simulink model "Rebuild"  (R2024b)
settings: Solver=VariableStepAuto  StartTime=0.0  StopTime=12  RelTol=1e-3
values from neighbouring files (symbols this model uses):
  A = 1.1    [RT14e_Parameters.m]    (also in RT15e_Parameters.m = 1.088; RT15evo_Parameters.m = 1.088)
  Aero_balance = 55    [RT14e_Parameters.m]    (also in RT15e_Parameters.m; RT15evo_Parameters.m)
  Aeromaps_ON = 0    [SIM_setup.m]
  air_density = 1.2    [SIM_setup.m]
  Balance_FW = Data_FW_STD(1:end,2)    [RT15e_Parameters.m]    (also in RT15evo_Parameters.m)
  Balance_R_11 = Data_R_11(1:end,2)    [RT15e_Parameters.m]    (also in RT15evo_Parameters.m)
  Br_coef_of_friction_F = 0.33    [RT14e_Parameters.m]    (also in RT15e_Parameters.m; RT15evo_Parameters.m)
  Br_coef_of_friction_R = 0.33    [RT14e_Parameters.m]    (also in RT15e_Parameters.m; RT15evo_Parameters.m)
  Br_pistons_area_F = 3617.26/1e6    (= 0.00361726)    [RT14e_Parameters.m]    (also in RT15e_Parameters.m; RT15evo_Parameters.m)
  Br_pistons_area_R = 2026.83/1e6    (= 0.00202683)    [RT14e_Parameters.m]    (also in RT15e_Parameters.m; RT15evo_Parameters.m)
  CdA = 1.31*A    (= 1.441)    [RT14e_Parameters.m]    (also in RT15e_Parameters.m = 1.700544; RT15evo_Parameters.m = 1.700544)
  CdA_FW = Data_FW_STD(1:end,3)    [RT15e_Parameters.m]    (also in RT15evo_Parameters.m)
  CdA_R_11 = Data_R_11(1:end,3)    [RT15e_Parameters.m]    (also in RT15evo_Parameters.m)
  ClA = 3.3*A    (= 3.63)    [RT14e_Parameters.m]    (also in RT15e_Parameters.m = 4.36288; RT15evo_Parameters.m = 4.36288)
  ClA_FW = Data_FW_STD(1:end,4)    [RT15e_Parameters.m]    (also in RT15evo_Parameters.m)
  ClA_R_11 = Data_R_11(1:end,4)    [RT15e_Parameters.m]    (also in RT15evo_Parameters.m)
  CoG_z = 0.35    [RT14e_Parameters.m]    (also in RT15e_Parameters.m = 0.28495; RT15evo_Parameters.m = 0.28495)
  Default_Fz_FL = Default_Fz_F/2 + (Default_Fz_F*CoG_y/Track_Front)    [RT14e_Parameters.m]    (also in RT15e_Parameters.m; RT15evo_Parameters.m)
  Default_Fz_FR = Default_Fz_F/2 - (Default_Fz_F*CoG_y/Track_Front)    [RT14e_Parameters.m]    (also in RT15e_Parameters.m; RT15evo_Parameters.m)
  Default_Fz_RL = Default_Fz_R/2 + (Default_Fz_R*CoG_y/Track_Rear)    [RT14e_Parameters.m]    (also in RT15e_Parameters.m; RT15evo_Parameters.m)
  Default_Fz_RR = Default_Fz_R/2 - (Default_Fz_R*CoG_y/Track_Rear)    [RT14e_Parameters.m]    (also in RT15e_Parameters.m; RT15evo_Parameters.m)
  Effective_br_disk_r_F = 0.0905    [RT14e_Parameters.m]    (also in RT15e_Parameters.m; RT15evo_Parameters.m)
  Effective_br_disk_r_R = 0.0895    [RT14e_Parameters.m]    (also in RT15e_Parameters.m; RT15evo_Parameters.m)
  Front_brake_balance = 0.0    (= 0)    [RT14e_Parameters.m]    (also in RT15e_Parameters.m; RT15evo_Parameters.m)
  Front_brake_pump_area = 153.94    [RT14e_Parameters.m]    (also in RT15e_Parameters.m; RT15evo_Parameters.m)
  Front_desired_brake_p_balance = 0.6    [RT14e_Parameters.m]    (also in RT15e_Parameters.m; RT15evo_Parameters.m)
  FW_Setup = Data_FW_STD(1:end,1)    [RT15e_Parameters.m]    (also in RT15evo_Parameters.m)
  Fx = Data_Fx(2:end,3:end)    [RT14e_Parameters.m]    (also in RT15e_Parameters.m; RT15evo_Parameters.m)
  Fy = Data_Fy(2:end,3:end)    [RT14e_Parameters.m]    (also in RT15e_Parameters.m; RT15evo_Parameters.m)
  Fz = Data_Fy(2:end,2)    [RT14e_Parameters.m]    (also in RT15e_Parameters.m; RT15evo_Parameters.m)
  g = 9.81    [SIM_setup.m]
  Gear_ratio = 12.9    [RT14e_Parameters.m]    (also in RT15e_Parameters.m; RT15evo_Parameters.m)
  Iz_wehicle = 120    [RT14e_Parameters.m]    (also in RT15e_Parameters.m; RT15evo_Parameters.m)
  Iz_wheel = 0.15    [RT14e_Parameters.m]    (also in RT15e_Parameters.m; RT15evo_Parameters.m)
  Lf = Wheelbase - CoG_x    (= 0.77)    [RT14e_Parameters.m]    (also in RT15e_Parameters.m = 0.7504; RT15evo_Parameters.m = 0.7504)
  LLTD = 0.45    [RT14e_Parameters.m]    (also in RT15e_Parameters.m = 0.55; RT15evo_Parameters.m = 0.55)
  Lock_brake_balance = false    [RT14e_Parameters.m]    (also in RT15e_Parameters.m; RT15evo_Parameters.m)
  Lr = Wheelbase - Lf    (= 0.755)    [RT14e_Parameters.m]    (also in RT15e_Parameters.m = 0.7746; RT15evo_Parameters.m = 0.7746)
  Mass = Vehicle_mass + Driver_mass    (= 290)    [RT14e_Parameters.m]    (also in RT15e_Parameters.m = 265; RT15evo_Parameters.m)
  Motor_maximum_power = 35366    [RT14e_Parameters.m]    (also in RT15e_Parameters.m; RT15evo_Parameters.m)
  RB_torque_setting_1 = -2    [RT14e_Parameters.m]    (also in RT15e_Parameters.m; RT15evo_Parameters.m)
  RB_torque_setting_10 = -20    [RT14e_Parameters.m]    (also in RT15e_Parameters.m; RT15evo_Parameters.m)
  RB_torque_setting_2 = -4    [RT14e_Parameters.m]    (also in RT15e_Parameters.m; RT15evo_Parameters.m)
  RB_torque_setting_3 = -6    [RT14e_Parameters.m]    (also in RT15e_Parameters.m; RT15evo_Parameters.m)
  RB_torque_setting_4 = -8    [RT14e_Parameters.m]    (also in RT15e_Parameters.m; RT15evo_Parameters.m)
  RB_torque_setting_5 = -10    [RT14e_Parameters.m]    (also in RT15e_Parameters.m; RT15evo_Parameters.m)
  RB_torque_setting_6 = -12    [RT14e_Parameters.m]    (also in RT15e_Parameters.m; RT15evo_Parameters.m)
  RB_torque_setting_7 = -14    [RT14e_Parameters.m]    (also in RT15e_Parameters.m; RT15evo_Parameters.m)
  RB_torque_setting_8 = -16    [RT14e_Parameters.m]    (also in RT15e_Parameters.m; RT15evo_Parameters.m)
  RB_torque_setting_9 = -18    [RT14e_Parameters.m]    (also in RT15e_Parameters.m; RT15evo_Parameters.m)
  Rear_brake_pump_area = 198.56    [RT14e_Parameters.m]    (also in RT15e_Parameters.m; RT15evo_Parameters.m)
  Roll_Angle_11 = Data_R_11(1:end,1)    [RT15e_Parameters.m]    (also in RT15evo_Parameters.m)
  SA = Data_Fy(1,3:end)    [RT14e_Parameters.m]    (also in RT15e_Parameters.m; RT15evo_Parameters.m)
  SR = Data_Fx(1,3:end)    [RT14e_Parameters.m]    (also in RT15e_Parameters.m; RT15evo_Parameters.m)
  start_acc_x = double(start_acc_x_ts.Data)    [SIM_setup.m]
  start_acc_y = double(start_acc_y_ts.Data)    [SIM_setup.m]
  start_time = 1188    [SIM_setup.m]
  start_velocity_x = double(start_velocity_x_ts.Data)    [SIM_setup.m]
  start_velocity_y = double(start_velocity_y_ts.Data)    [SIM_setup.m]
  start_yaw_acc = double(start_yaw_acc_ts.Data)    [SIM_setup.m]
  start_yaw_rate = double(start_yaw_rate_ts.Data)    [SIM_setup.m]
  Static_Camber_FL = 0    [RT14e_Parameters.m]    (also in RT15e_Parameters.m; RT15evo_Parameters.m)
  Static_Camber_FR = 0    [RT14e_Parameters.m]    (also in RT15e_Parameters.m; RT15evo_Parameters.m)
  Static_Camber_RL = 0    [RT14e_Parameters.m]    (also in RT15e_Parameters.m; RT15evo_Parameters.m)
  Static_Camber_RR = 0    [RT14e_Parameters.m]    (also in RT15e_Parameters.m; RT15evo_Parameters.m)
  Static_Toe_FL = 0    [RT14e_Parameters.m]    (also in RT15e_Parameters.m; RT15evo_Parameters.m)
  Static_Toe_FR = 0    [RT14e_Parameters.m]    (also in RT15e_Parameters.m; RT15evo_Parameters.m)
  Static_Toe_RL = 0    [RT14e_Parameters.m]    (also in RT15e_Parameters.m; RT15evo_Parameters.m)
  Static_Toe_RR = 0    [RT14e_Parameters.m]    (also in RT15e_Parameters.m; RT15evo_Parameters.m)
  Steering_Angle_FL = Data_Steering(1:end,2)    [RT14e_Parameters.m]    (also in RT15e_Parameters.m; RT15evo_Parameters.m)
  Steering_Angle_FR = Data_Steering(1:end,3)    [RT14e_Parameters.m]    (also in RT15e_Parameters.m; RT15evo_Parameters.m)
  Steering_Wheel_Angle = Data_Steering(1:end,1)    [RT14e_Parameters.m]    (also in RT15e_Parameters.m; RT15evo_Parameters.m)
  Tire_radius = 0.203    [RT14e_Parameters.m]    (also in RT15e_Parameters.m; RT15evo_Parameters.m)
  Torque_limit_2 = Motor_maximum_torque*0.2    (= 5.82)    [RT14e_Parameters.m]    (also in RT15e_Parameters.m; RT15evo_Parameters.m)
  Torque_limit_3 = Motor_maximum_torque*0.3    (= 8.73)    [RT14e_Parameters.m]    (also in RT15e_Parameters.m; RT15evo_Parameters.m)
  Torque_limit_4 = Motor_maximum_torque*0.4    (= 11.64)    [RT14e_Parameters.m]    (also in RT15e_Parameters.m; RT15evo_Parameters.m)
  Torque_limit_5 = Motor_maximum_torque*0.5    (= 14.55)    [RT14e_Parameters.m]    (also in RT15e_Parameters.m; RT15evo_Parameters.m)
  Torque_limit_6 = Motor_maximum_torque*0.6    (= 17.46)    [RT14e_Parameters.m]    (also in RT15e_Parameters.m; RT15evo_Parameters.m)
  Torque_limit_7 = Motor_maximum_torque*0.7    (= 20.37)    [RT14e_Parameters.m]    (also in RT15e_Parameters.m; RT15evo_Parameters.m)
  Torque_limit_8 = Motor_maximum_torque*0.8    (= 23.28)    [RT14e_Parameters.m]    (also in RT15e_Parameters.m; RT15evo_Parameters.m)
  Torque_limit_9 = 29.1    [RT14e_Parameters.m]    (also in RT15e_Parameters.m; RT15evo_Parameters.m)
  Torque_limit_max = Motor_maximum_torque    (= 29.1)    [RT14e_Parameters.m]    (also in RT15e_Parameters.m; RT15evo_Parameters.m)
  Torque_limit_min = Motor_maximum_torque*0.1    (= 2.91)    [RT14e_Parameters.m]    (also in RT15e_Parameters.m; RT15evo_Parameters.m)
  Torque_limit_set = 10    [RT14e_Parameters.m]    (also in RT15e_Parameters.m; RT15evo_Parameters.m)
  Track_Front = 1.2    [RT14e_Parameters.m]    (also in RT15e_Parameters.m; RT15evo_Parameters.m)
  Track_Rear = 1.18    [RT14e_Parameters.m]    (also in RT15e_Parameters.m; RT15evo_Parameters.m)
  TV_ON = 0    [SIM_setup.m]
  TV_RB_understeer_gradient_1 = -0.5    [RT14e_Parameters.m]    (also in RT15e_Parameters.m; RT15evo_Parameters.m)
  TV_RB_understeer_gradient_10 = 0.005    [RT14e_Parameters.m]    (also in RT15e_Parameters.m; RT15evo_Parameters.m)
  TV_RB_understeer_gradient_2 = -0.1    [RT14e_Parameters.m]    (also in RT15e_Parameters.m; RT15evo_Parameters.m)
  TV_RB_understeer_gradient_3 = 0.08    [RT14e_Parameters.m]    (also in RT15e_Parameters.m; RT15evo_Parameters.m)
  TV_RB_understeer_gradient_4 = 0.06    [RT14e_Parameters.m]    (also in RT15e_Parameters.m; RT15evo_Parameters.m)
  TV_RB_understeer_gradient_5 = 0.05    [RT14e_Parameters.m]    (also in RT15e_Parameters.m; RT15evo_Parameters.m)
  TV_RB_understeer_gradient_6 = 0.04    [RT14e_Parameters.m]    (also in RT15e_Parameters.m; RT15evo_Parameters.m)
  TV_RB_understeer_gradient_7 = 0.03    [RT14e_Parameters.m]    (also in RT15e_Parameters.m; RT15evo_Parameters.m)
  TV_RB_understeer_gradient_8 = 0.02    [RT14e_Parameters.m]    (also in RT15e_Parameters.m; RT15evo_Parameters.m)
  TV_RB_understeer_gradient_9 = 0.01    [RT14e_Parameters.m]    (also in RT15e_Parameters.m; RT15evo_Parameters.m)
  TV_understeer_gradient_1 = -0.5    [RT14e_Parameters.m]    (also in RT15e_Parameters.m; RT15evo_Parameters.m)
  TV_understeer_gradient_10 = 0.002    [RT14e_Parameters.m]    (also in RT15e_Parameters.m; RT15evo_Parameters.m)
  TV_understeer_gradient_2 = -0.1    [RT14e_Parameters.m]    (also in RT15e_Parameters.m; RT15evo_Parameters.m)
  TV_understeer_gradient_3 = 0.06    [RT14e_Parameters.m]    (also in RT15e_Parameters.m; RT15evo_Parameters.m)
  TV_understeer_gradient_4 = 0.05    [RT14e_Parameters.m]    (also in RT15e_Parameters.m; RT15evo_Parameters.m)
  TV_understeer_gradient_5 = 0.04    [RT14e_Parameters.m]    (also in RT15e_Parameters.m; RT15evo_Parameters.m)
  TV_understeer_gradient_6 = 0.03    [RT14e_Parameters.m]    (also in RT15e_Parameters.m; RT15evo_Parameters.m)
  TV_understeer_gradient_7 = 0.02    [RT14e_Parameters.m]    (also in RT15e_Parameters.m; RT15evo_Parameters.m)
  TV_understeer_gradient_8 = 0.01    [RT14e_Parameters.m]    (also in RT15e_Parameters.m; RT15evo_Parameters.m)
  TV_understeer_gradient_9 = 0.005    [RT14e_Parameters.m]    (also in RT15e_Parameters.m; RT15evo_Parameters.m)
  Vx_APPS_ON = 1    [SIM_setup.m]
  Wheel_rolling_resistance = 0.055    [RT14e_Parameters.m]    (also in RT15e_Parameters.m; RT15evo_Parameters.m)
  Wheelbase = 1.525    [RT14e_Parameters.m]    (also in RT15e_Parameters.m; RT15evo_Parameters.m)
undefined symbols (not defined in the file or in its folder): Actual_Torque_Value_RL, Actual_Torque_Value_RR, aero_balance, APPS, Brake_Pressure_Front, Brake_Pressure_Rear, Cl, lateral_load_transfer_distribution, maths_GPS_Velocity, Max_Torque, rad, s, Steering_position, tire_radius, wheel_base, Wheel_Speed_RL, Wheel_Speed_RR, Xsens_MTI_670_accX, Xsens_MTI_670_accY, Xsens_MTI_670_gyrZ
libraries: simulink x30, simulink_extras x11, slpidlib x9, dspstat3 x4, slrealtimeloglib x1, aerolibconvert2 x1
(part 2 of 6)

== system Rebuild/Main/Wheels & Tires/Fx ==
  Slips : Inport
  2-D Lookup Table1 : Lookup_n-D  BreakpointsForDimension1=Fz  BreakpointsForDimension2=SR  Table=Fx  UseLastTableValue=on  ApplyAccurateEfficientRounding=on  InternalRulePriority=Speed  RndMeth=Simplest
      settings: InputPortMap=u0,u1
  2-D Lookup Table2 : Lookup_n-D  BreakpointsForDimension1=Fz  BreakpointsForDimension2=SR  Table=Fx  UseLastTableValue=on  ApplyAccurateEfficientRounding=on  InternalRulePriority=Speed  RndMeth=Simplest
      settings: InputPortMap=u0,u1
  2-D Lookup Table3 : Lookup_n-D  BreakpointsForDimension1=Fz  BreakpointsForDimension2=SR  Table=Fx  ExtrapMethod=Clip  UseLastTableValue=on  ApplyAccurateEfficientRounding=on  InternalRulePriority=Speed  RndMeth=Simplest
      settings: InputPortMap=u0,u1
  2-D Lookup Table4 : Lookup_n-D  BreakpointsForDimension1=Fz  BreakpointsForDimension2=SR  Table=Fx  ExtrapMethod=Clip  UseLastTableValue=on  ApplyAccurateEfficientRounding=on  InternalRulePriority=Speed  RndMeth=Simplest
      settings: InputPortMap=u0,u1
  Bus Creator : BusCreator  Inputs=4
  Bus Selector : BusSelector  OutputSignals=Slip Ratio.Slip Ratio FL
  Bus Selector1 : BusSelector  OutputSignals=Tire Forces [N[.Fz [N].Fz FL [N]
  Bus Selector2 : BusSelector  OutputSignals=Slip Ratio.Slip Ratio FR
  Bus Selector3 : BusSelector  OutputSignals=Tire Forces [N[.Fz [N].Fz FR [N]
  Bus Selector4 : BusSelector  OutputSignals=Slip Ratio.Slip Ratio RL
  Bus Selector5 : BusSelector  OutputSignals=Tire Forces [N[.Fz [N].Fz RL [N]
  Bus Selector6 : BusSelector  OutputSignals=Slip Ratio.Slip Ratio RR
  Bus Selector7 : BusSelector  OutputSignals=Tire Forces [N[.Fz [N].Fz RR [N]
  Gain{,1..3} (4 alike) : Gain
  Fx [N] : Outport
  wires:
  2-D Lookup Table1/1 -> Gain/1  "Fx FL [N]"
  2-D Lookup Table2/1 -> Gain1/1  "Fx FR [N]"
  2-D Lookup Table3/1 -> Gain2/1  "Fx RL [N]"
  2-D Lookup Table4/1 -> Gain3/1  "Fx RR [N]"
  Bus Creator/1 -> Fx [N]/1  "Fx [N]"
  Slips/1 -> Bus Selector/1, Bus Selector6/1, Bus Selector4/1, Bus Selector2/1
  [Tires] -> Bus Selector1/1, Bus Selector7/1, Bus Selector5/1, Bus Selector3/1
  Bus Selector/1 -> 2-D Lookup Table1/2  "<Slip Ratio FL>"
  Bus Selector1/1 -> 2-D Lookup Table1/1  "<Fz FL [N]>"
  Bus Selector3/1 -> 2-D Lookup Table2/1  "<Fz FR [N]>"
  Bus Selector2/1 -> 2-D Lookup Table2/2  "<Slip Ratio FR>"
  Bus Selector5/1 -> 2-D Lookup Table3/1  "<Fz RL [N]>"
  Bus Selector4/1 -> 2-D Lookup Table3/2  "<Slip Ratio RL>"
  Bus Selector7/1 -> 2-D Lookup Table4/1  "<Fz RR [N]>"
  Bus Selector6/1 -> 2-D Lookup Table4/2  "<Slip Ratio RR>"
  Gain/1 -> Bus Creator/1  "Fx FL [N]"
  Gain1/1 -> Bus Creator/2  "Fx FR [N]"
  Gain2/1 -> Bus Creator/3  "Fx RL [N]"
  Gain3/1 -> Bus Creator/4  "Fx RR [N]"

== system Rebuild/Main/Wheels & Tires/Fy ==
  Slips : Inport
  2-D Lookup Table{,1..3} (4 alike) : Lookup_n-D  BreakpointsForDimension1=Fz  BreakpointsForDimension2=SA  Table=Fy  ExtrapMethod=Clip  UseLastTableValue=on  ApplyAccurateEfficientRounding=on  InternalRulePriority=Speed  RndMeth=Simplest
      settings: InputPortMap=u0,u1
  Bus Creator : BusCreator  Inputs=4
  Bus Selector : BusSelector  OutputSignals=Slip Angle [deg].Slip Angle FL [deg]
  Bus Selector1 : BusSelector  OutputSignals=Tire Forces [N[.Fz [N].Fz FL [N]
  Bus Selector2 : BusSelector  OutputSignals=Slip Angle [deg].Slip Angle FR [deg]
  Bus Selector3 : BusSelector  OutputSignals=Tire Forces [N[.Fz [N].Fz FR [N]
  Bus Selector4 : BusSelector  OutputSignals=Slip Angle [deg].Slip Angle RL [deg]
  Bus Selector5 : BusSelector  OutputSignals=Tire Forces [N[.Fz [N].Fz RL [N]
  Bus Selector6 : BusSelector  OutputSignals=Slip Angle [deg].Slip Angle RR [deg]
  Bus Selector7 : BusSelector  OutputSignals=Tire Forces [N[.Fz [N].Fz RR [N]
  Gain{,1..3} (4 alike) : Gain
  Fy [N] : Outport
  wires:
  2-D Lookup Table/1 -> Gain3/1  "Fy FL [N]"
  2-D Lookup Table1/1 -> Gain2/1  "Fy FR [N]"
  2-D Lookup Table3/1 -> Gain1/1  "Fy RL [N]"
  2-D Lookup Table2/1 -> Gain/1  "Fy RR [N]"
  Bus Creator/1 -> Fy [N]/1  "Fy [N]"
  Bus Selector2/1 -> 2-D Lookup Table1/2  "<Slip Angle FR [deg]>"
  Bus Selector3/1 -> 2-D Lookup Table1/1  "<Fz FR [N]>"
  Bus Selector/1 -> 2-D Lookup Table/2  "<Slip Angle FL [deg]>"
  Slips/1 -> Bus Selector/1, Bus Selector6/1, Bus Selector4/1, Bus Selector2/1
  [Tires] -> Bus Selector1/1, Bus Selector7/1, Bus Selector5/1, Bus Selector3/1
  Bus Selector1/1 -> 2-D Lookup Table/1  "<Fz FL [N]>"
  Bus Selector6/1 -> 2-D Lookup Table2/2  "<Slip Angle RR [deg]>"
  Bus Selector7/1 -> 2-D Lookup Table2/1  "<Fz RR [N]>"
  Bus Selector4/1 -> 2-D Lookup Table3/2  "<Slip Angle RL [deg]>"
  Bus Selector5/1 -> 2-D Lookup Table3/1  "<Fz RL [N]>"
  Gain/1 -> Bus Creator/4  "Fy RR [N]"
  Gain1/1 -> Bus Creator/3  "Fy RL [N]"
  Gain2/1 -> Bus Creator/2  "Fy FR [N]"
  Gain3/1 -> Bus Creator/1  "Fy FL [N]"

== system Rebuild/Main/Wheels & Tires/Fz ==
  Add{,1..3} (4 alike) : Sum  Inputs=+++
  Bus Creator : BusCreator  Inputs=4
  Bus Selector : BusSelector  OutputSignals=Aero Wheel Loads [N].Aero Load FL [N]
  Bus Selector1 : BusSelector  OutputSignals=Load Transfer [N].Wheel Load Transfer [N].Load Transfer FL [N]
  Bus Selector2 : BusSelector  OutputSignals=Aero Wheel Loads [N].Aero Load FR [N]
  Bus Selector3 : BusSelector  OutputSignals=Load Transfer [N].Wheel Load Transfer [N].Load Transfer FR [N]
  Bus Selector4 : BusSelector  OutputSignals=Aero Wheel Loads [N].Aero Load RL [N]
  Bus Selector5 : BusSelector  OutputSignals=Load Transfer [N].Wheel Load Transfer [N].Load Transfer RL [N]
  Bus Selector6 : BusSelector  OutputSignals=Aero Wheel Loads [N].Aero Load RR [N]
  Bus Selector7 : BusSelector  OutputSignals=Load Transfer [N].Wheel Load Transfer [N].Load Transfer RR [N]
  Constant1 : Constant  Value=Default_Fz_FR
  Constant2 : Constant  Value=Default_Fz_RL
  Constant3 : Constant  Value=Default_Fz_RR
  Constant5 : Constant  Value=Default_Fz_FL
  Fz [N] : Outport
  wires:
  Add3/1 -> Bus Creator/4  "Fz RR [N]"
  Add2/1 -> Bus Creator/3  "Fz RL [N]"
  Add1/1 -> Bus Creator/2  "Fz FR [N]"
  Add/1 -> Bus Creator/1  "Fz FL [N]"
  Bus Creator/1 -> Fz [N]/1  "Fz [N]"
  Constant5/1 -> Add/3
  Constant1/1 -> Add1/3
  Constant2/1 -> Add2/3
  Constant3/1 -> Add3/3
  [Sus] -> Bus Selector7/1, Bus Selector5/1, Bus Selector3/1, Bus Selector1/1
  Bus Selector/1 -> Add/1  "<Aero Load FL [N]>"
  Bus Selector1/1 -> Add/2  "<Load Transfer FL [N]>"
  Bus Selector3/1 -> Add1/2  "<Load Transfer FR [N]>"
  Bus Selector2/1 -> Add1/1  "<Aero Load FR [N]>"
  [Aero] -> Bus Selector6/1, Bus Selector4/1, Bus Selector2/1, Bus Selector/1
  Bus Selector6/1 -> Add3/1  "<Aero Load RR [N]>"
  Bus Selector7/1 -> Add3/2  "<Load Transfer RR [N]>"
  Bus Selector4/1 -> Add2/1  "<Aero Load RL [N]>"
  Bus Selector5/1 -> Add2/2  "<Load Transfer RL [N]>"

== system Rebuild/Main/Wheels & Tires/Slip Ratio & Slip Angle Calculation ==
  Wheel Speeds [rad/s] : Inport
  Bus Creator : BusCreator  Inputs=4
  Bus Creator1 : BusCreator  Inputs=4
  Bus Selector : BusSelector  Commented=on  OutputSignals=Slip Angle FL [rad],Slip Angle FR [rad],Slip Angle RL [rad],Slip Angle RR [rad]
  Bus Selector1 : BusSelector  Commented=on  OutputSignals=Slip Ratio FL,Slip Ratio FR,Slip Ratio RL,Slip Ratio RR
  Bus Selector2 : BusSelector  OutputSignals=Slip Angle FL [rad],Slip Angle FR [rad],Slip Angle RL [rad],Slip Angle RR [rad]
  Clock : Clock  Commented=on
  Radians to Degrees{1..4} (4 alike) : simulink_extras/Transformations/Radians to Degrees
  Saturation : Saturate  Commented=on  UpperLimit=0.2  LowerLimit=-0.2
  Saturation1 : Saturate  Commented=on  UpperLimit=0.05  LowerLimit=-0.05
  Saturation{3,5..7} (4 alike) : Saturate  UpperLimit=0.35  LowerLimit=-0.35
  Slip Angle : Subsystem
  "Slip Ratio " : Subsystem
  Switch : Switch  Commented=on  Criteria=u2 > Threshold  Threshold=0.2  SaturateOnIntegerOverflow=off  InputSameDT=off
  Slip Ratio : Outport
  Slip Angles [deg] : Outport  Port=2
  wires:
  "Slip Ratio "/1(Slip Ratio) -> Slip Ratio/1  "Slip Ratio"
  Wheel Speeds [rad/s]/1 -> "Slip Ratio "/1(Wheel Speeds [rad/s])
  ? -> ?
  Saturation1/1 -> Switch/3
  Saturation/1 -> Switch/1
  Clock/1 -> Switch/2
  Switch/1 -> ?
  Slip Angle/1(Slip Angle [rad]) -> Bus Selector2/1  "Slip Angles"
  Bus Selector2/1 -> Saturation3/1  "<Slip Angle FL [rad]>"
  Bus Selector2/2 -> Saturation5/1  "<Slip Angle FR [rad]>"
  Bus Selector2/3 -> Saturation6/1  "<Slip Angle RL [rad]>"
  Bus Selector2/4 -> Saturation7/1  "<Slip Angle RR [rad]>"
  Radians to Degrees2/1 -> Bus Creator1/2  "Slip Angle FR [deg]"
  Radians to Degrees1/1 -> Bus Creator1/1  "Slip Angle FL [deg]"
  Radians to Degrees3/1 -> Bus Creator1/3  "Slip Angle RL [deg]"
  Radians to Degrees4/1 -> Bus Creator1/4  "Slip Angle RR [deg]"
  Bus Creator1/1 -> Slip Angles [deg]/1  "Slip Angles"
  Saturation3/1 -> Radians to Degrees1/1
  Saturation5/1 -> Radians to Degrees2/1
  Saturation6/1 -> Radians to Degrees3/1
  Saturation7/1 -> Radians to Degrees4/1

== system Rebuild/Main/Wheels & Tires/Wheel Speeds ==
  Motor Torque [Nm] : Inport
  Fx [N] : Inport  Port=2
  Fz [N] : Inport  Port=3
  Brake Torque [Nm] : Inport  Port=4
  Angular Velocity Conversion : aerolibconvert2/Angular Velocity Conversion  IU=rad/s  OU=rpm
  Bus Creator : BusCreator  Inputs=4
  Bus Creator1 : BusCreator  Inputs=2
  Bus Creator2 : BusCreator  Inputs=2
  Rolling Resistance Calculation : Subsystem
  Wheel Speed FL : Subsystem
  Wheel Speed FR : Subsystem
  Wheel Speed RL : Subsystem
  Wheel Speed RR : Subsystem
  Wheel Speeds : Outport
  wires:
  Fx [N]/1 -> Wheel Speed RR/2(Fx [N]), Wheel Speed RL/2(Fx [N]), Wheel Speed FR/2(Fx [N]), Wheel Speed FL/2(Fx [N])
  Bus Creator/1 -> Bus Creator2/1, Angular Velocity Conversion/1  "Wheel Speeds [rad/s]"
  Wheel Speed FR/1(Wheel Speed FR [rad/s]) -> Bus Creator/2  "Wheel Speed FR [rad/s]"
  Wheel Speed FL/1(Wheel Speed FL [rad/s]) -> Bus Creator/1  "Wheel Speed FL [rad/s]"
  Wheel Speed RL/1(Wheel Speed RL [rad/s]) -> Bus Creator/3  "Wheel Speed RL [rad/s]"
  Wheel Speed RR/1(Wheel Speed RL [rad/s]) -> Bus Creator/4  "Wheel Speed RR [rad/s]"
  Fz [N]/1 -> Rolling Resistance Calculation/1(Fz [N])
  Motor Torque [Nm]/1 -> Bus Creator1/2
  Brake Torque [Nm]/1 -> Bus Creator1/1
  Rolling Resistance Calculation/1(Rolling Resistance) -> Wheel Speed RR/1(Rolling Resistance), Wheel Speed RL/1(Rolling Resistance), Wheel Speed FR/1(Rolling Resistance), Wheel Speed FL/1(Rolling Resistance)
  Bus Creator1/1 -> Wheel Speed RR/3(Torque [Nm]), Wheel Speed RL/3(Torque [Nm]), Wheel Speed FR/3(Torque [Nm]), Wheel Speed FL/3(Torque [Nm])  "Torque [Nm]"
  Angular Velocity Conversion/1 -> Bus Creator2/2  "Wheel Speeds [rpm]"
  Bus Creator2/1 -> Wheel Speeds/1  "Wheel Speeds"

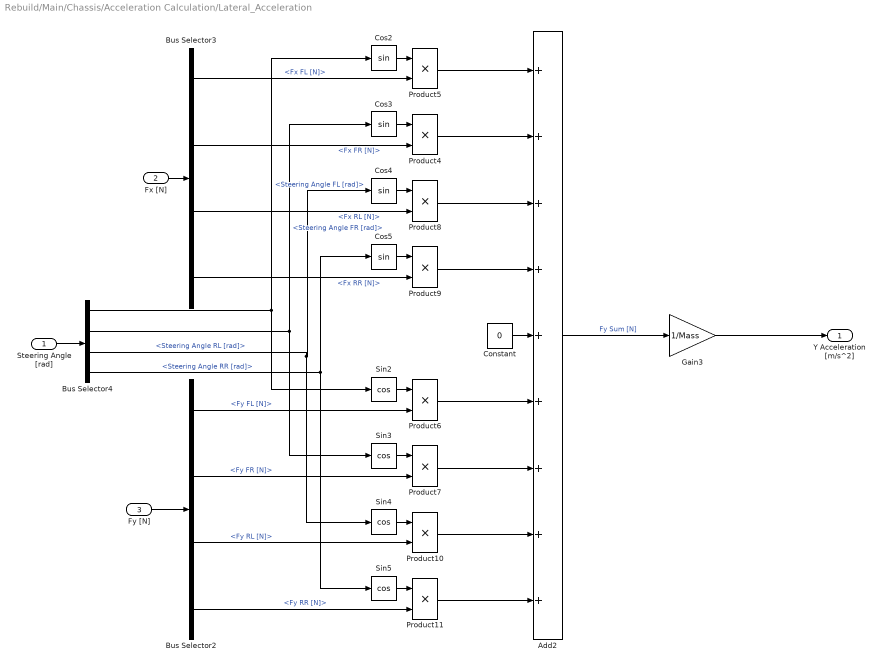
== system Rebuild/Main/Chassis/Acceleration Calculation/Lateral_Acceleration ==
  Steering Angle [rad] : Inport
  Fx [N] : Inport  Port=2
  Fy [N] : Inport  Port=3
  Add2 : Sum  Inputs=+++++++++
  Bus Selector2 : BusSelector  OutputSignals=Fy FL [N],Fy FR [N],Fy RL [N],Fy RR [N]
  Bus Selector3 : BusSelector  OutputSignals=Fx FL [N],Fx FR [N],Fx RL [N],Fx RR [N]
  Bus Selector4 : BusSelector  OutputSignals=Steering Angle FL [rad],Steering Angle FR [rad],Steering Angle RL [rad],Steering Angle RR [rad]
  Constant : Constant  Value=0
  Cos{2..5} (4 alike) : Trigonometry
  Gain3 : Gain  Gain=1/Mass
  Product{4..11} (8 alike) : Product
  Sin{2..5} (4 alike) : Trigonometry  Operator=cos
  Y Acceleration [m/s^2] : Outport
  wires:
  Bus Selector4/3 -> Sin4/1, Cos4/1  "<Steering Angle RL [rad]>"
  Steering Angle [rad]/1 -> Bus Selector4/1
  Bus Selector4/4 -> Sin5/1, Cos5/1  "<Steering Angle RR [rad]>"
  Bus Selector3/1 -> Product5/2  "<Fx FL [N]>"
  Gain3/1 -> Y Acceleration [m/s^2]/1
  Add2/1 -> Gain3/1  "Fy Sum [N]"
  Product4/1 -> Add2/2
  Fy [N]/1 -> Bus Selector2/1
  Bus Selector4/1 -> Sin2/1, Cos2/1  "<Steering Angle FL [rad]>"
  Fx [N]/1 -> Bus Selector3/1
  Cos2/1 -> Product5/1
  Product5/1 -> Add2/1
  Product7/1 -> Add2/7
  Product6/1 -> Add2/6
  Cos3/1 -> Product4/1
  Sin2/1 -> Product6/1
  Sin3/1 -> Product7/1
  Sin4/1 -> Product10/1
  Bus Selector3/2 -> Product4/2  "<Fx FR [N]>"
  Cos5/1 -> Product9/1
  Bus Selector4/2 -> Sin3/1, Cos3/1  "<Steering Angle FR [rad]>"
  Cos4/1 -> Product8/1
  Bus Selector2/2 -> Product7/2  "<Fy FR [N]>"
  Sin5/1 -> Product11/1
  Bus Selector2/1 -> Product6/2  "<Fy FL [N]>"
  Constant/1 -> Add2/5
  Bus Selector3/3 -> Product8/2  "<Fx RL [N]>"
  Bus Selector3/4 -> Product9/2  "<Fx RR [N]>"
  Product8/1 -> Add2/3
  Product9/1 -> Add2/4
  Bus Selector2/3 -> Product10/2  "<Fy RL [N]>"
  Product10/1 -> Add2/8
  Bus Selector2/4 -> Product11/2  "<Fy RR [N]>"
  Product11/1 -> Add2/9

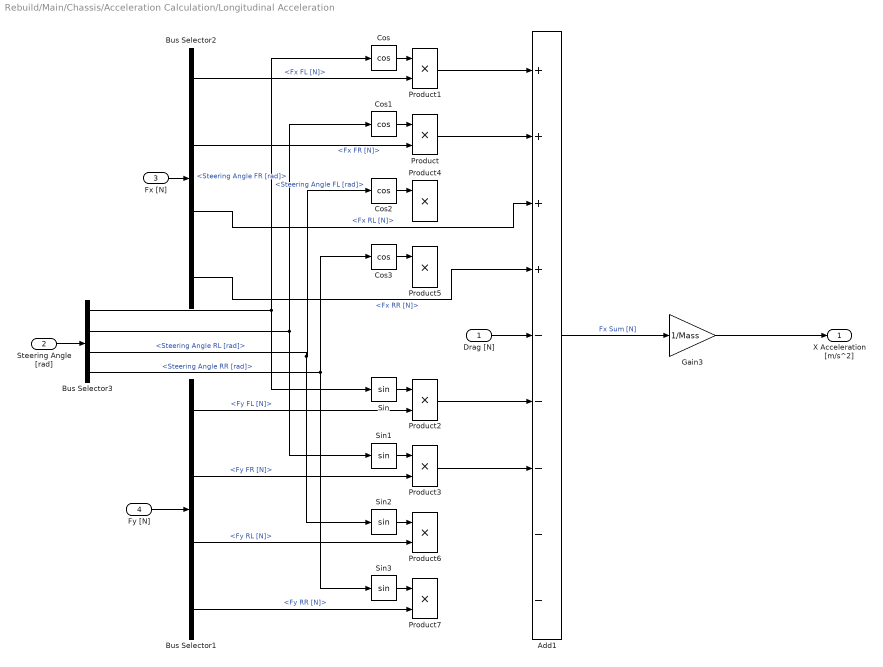
== system Rebuild/Main/Chassis/Acceleration Calculation/Longitudinal Acceleration ==
  Drag [N] : Inport
  Steering Angle [rad] : Inport  Port=2
  Fx [N] : Inport  Port=3
  Fy [N] : Inport  Port=4
  Add1 : Sum  Inputs=++++-----
  Bus Selector1 : BusSelector  OutputSignals=Fy FL [N],Fy FR [N],Fy RL [N],Fy RR [N]
  Bus Selector2 : BusSelector  OutputSignals=Fx FL [N],Fx FR [N],Fx RL [N],Fx RR [N]
  Bus Selector3 : BusSelector  OutputSignals=Steering Angle FL [rad],Steering Angle FR [rad],Steering Angle RL [rad],Steering Angle RR [rad]
  Cos{,1..3} (4 alike) : Trigonometry  Operator=cos
  Gain3 : Gain  Gain=1/Mass
  Product{,1..7} (8 alike) : Product
  Sin{,1..3} (4 alike) : Trigonometry
  X Acceleration [m/s^2] : Outport
  wires:
  Steering Angle [rad]/1 -> Bus Selector3/1
  Fx [N]/1 -> Bus Selector2/1
  Product/1 -> Add1/2
  Cos1/1 -> Product/1
  Cos/1 -> Product1/1
  Product1/1 -> Add1/1
  Fy [N]/1 -> Bus Selector1/1
  Bus Selector2/1 -> Product1/2  "<Fx FL [N]>"
  Bus Selector2/2 -> Product/2  "<Fx FR [N]>"
  Add1/1 -> Gain3/1  "Fx Sum [N]"
  Gain3/1 -> X Acceleration [m/s^2]/1
  Bus Selector3/1 -> Sin/1, Cos/1  "<Steering Angle FL [rad]>"
  Bus Selector3/2 -> Sin1/1, Cos1/1  "<Steering Angle FR [rad]>"
  Bus Selector3/3 -> Sin2/1, Cos2/1  "<Steering Angle RL [rad]>"
  Bus Selector3/4 -> Sin3/1, Cos3/1  "<Steering Angle RR [rad]>"
  Bus Selector2/3 -> Add1/3  "<Fx RL [N]>"
  Bus Selector2/4 -> Add1/4  "<Fx RR [N]>"
  Cos2/1 -> Product4/1
  Cos3/1 -> Product5/1
  Drag [N]/1 -> Add1/5
  Sin/1 -> Product2/1
  Bus Selector1/1 -> Product2/2  "<Fy FL [N]>"
  Sin1/1 -> Product3/1
  Bus Selector1/2 -> Product3/2  "<Fy FR [N]>"
  Bus Selector1/4 -> Product7/2  "<Fy RR [N]>"
  Sin3/1 -> Product7/1
  Bus Selector1/3 -> Product6/2  "<Fy RL [N]>"
  Sin2/1 -> Product6/1
  Product2/1 -> Add1/6
  Product3/1 -> Add1/7

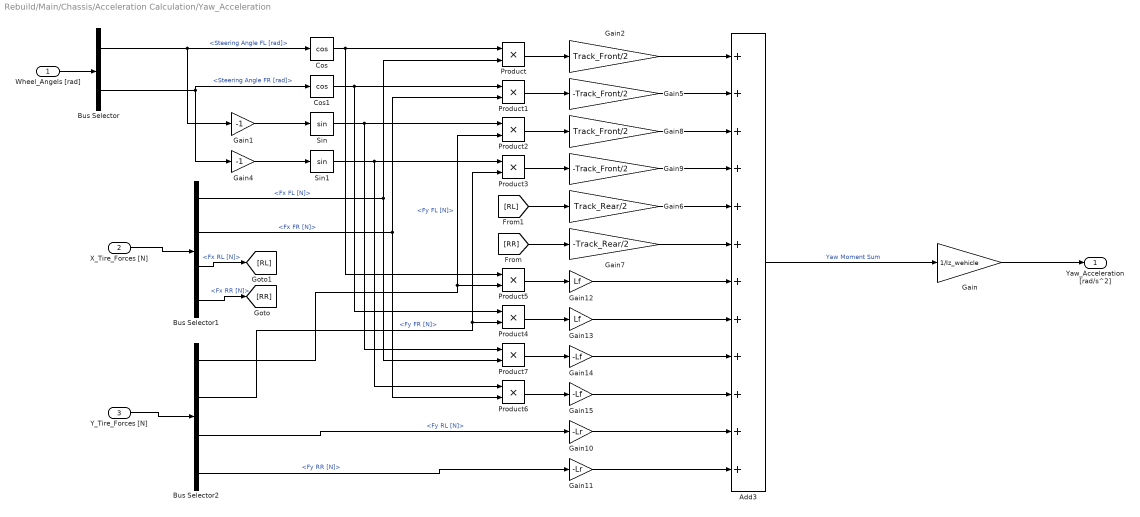
== system Rebuild/Main/Chassis/Acceleration Calculation/Yaw_Acceleration ==
  Wheel_Angels [rad] : Inport
  X_Tire_Forces [N] : Inport  Port=2
  Y_Tire_Forces [N] : Inport  Port=3
  Add3 : Sum  Inputs=++++++++++++
  Bus Selector : BusSelector  OutputSignals=Steering Angle FL [rad],Steering Angle FR [rad]
  Bus Selector1 : BusSelector  OutputSignals=Fx FL [N],Fx FR [N],Fx RL [N],Fx RR [N]
  Bus Selector2 : BusSelector  OutputSignals=Fy FL [N],Fy FR [N],Fy RL [N],Fy RR [N]
  Cos : Trigonometry  Operator=cos
  Cos1 : Trigonometry  Operator=cos
  Gain : Gain  Gain=1/Iz_wehicle
  Gain1 : Gain  Gain=-1
  Gain10 : Gain  Gain=-Lr
  Gain11 : Gain  Gain=-Lr
  Gain12 : Gain  Gain=Lf
  Gain13 : Gain  Gain=Lf
  Gain14 : Gain  Gain=-Lf
  Gain15 : Gain  Gain=-Lf
  Gain2 : Gain  Gain=Track_Front/2
  Gain4 : Gain  Gain=-1
  Gain5 : Gain  Gain=-Track_Front/2
  Gain6 : Gain  Gain=Track_Rear/2
  Gain7 : Gain  Gain=-Track_Rear/2
  Gain8 : Gain  Gain=Track_Front/2
  Gain9 : Gain  Gain=-Track_Front/2
  Product{,1..7} (8 alike) : Product
  Sin : Trigonometry
  Sin1 : Trigonometry
  Yaw_Acceleration [rad/s^2] : Outport
  wires:
  Add3/1 -> Gain/1  "Yaw Moment Sum"
  Gain/1 -> Yaw_Acceleration [rad/s^2]/1
  Gain4/1 -> Sin1/1
  Wheel_Angels [rad]/1 -> Bus Selector/1
  Gain1/1 -> Sin/1
  Bus Selector/1 -> Gain1/1, Cos/1  "<Steering Angle FL [rad]>"
  Bus Selector/2 -> Cos1/1, Gain4/1  "<Steering Angle FR [rad]>"
  Y_Tire_Forces [N]/1 -> Bus Selector2/1
  Cos/1 -> Product/1, Product5/1
  Cos1/1 -> Product1/1, Product4/1
  Product/1 -> Gain2/1
  Product1/1 -> Gain5/1
  Sin/1 -> Product2/1, Product7/1
  Product2/1 -> Gain8/1
  Sin1/1 -> Product3/1, Product6/1
  Product5/1 -> Gain12/1
  Product4/1 -> Gain13/1
  Product6/1 -> Gain15/1
  Product7/1 -> Gain14/1
  X_Tire_Forces [N]/1 -> Bus Selector1/1
  Bus Selector1/2 -> Product1/2, Product6/2  "<Fx FR [N]>"
  Bus Selector1/1 -> Product/2, Product7/2  "<Fx FL [N]>"
  Bus Selector2/2 -> Product4/2, Product3/2  "<Fy FR [N]>"
  Bus Selector2/1 -> Product5/2, Product2/2  "<Fy FL [N]>"
  Gain2/1 -> Add3/1
  Gain5/1 -> Add3/2
  Gain6/1 -> Add3/5
  Gain7/1 -> Add3/6
  Gain8/1 -> Add3/3
  Gain9/1 -> Add3/4
  Product3/1 -> Gain9/1
  Bus Selector2/3 -> Gain10/1  "<Fy RL [N]>"
  Gain10/1 -> Add3/11
  Gain11/1 -> Add3/12
  Bus Selector2/4 -> Gain11/1  "<Fy RR [N]>"
  Gain12/1 -> Add3/7
  Gain13/1 -> Add3/8
  Gain14/1 -> Add3/9
  Gain15/1 -> Add3/10
  [RR] -> Gain7/1
  Bus Selector1/4 -> [RR]  "<Fx RR [N]>"
  [RL] -> Gain6/1
  Bus Selector1/3 -> [RL]  "<Fx RL [N]>"

== system Rebuild/Main/Powertrain/Motors/Control Algorithms ==
  Motor Torque after FW [Nm] : Inport
  ABS : Subsystem  Commented=on
  ABS1 : Subsystem  Commented=on
  Bus Creator : BusCreator  Inputs=4
  Bus Selector : BusSelector  OutputSignals=Motor Torque FL after FW [Nm],Motor Torque FR after FW [Nm],Motor Torque RL after FW [Nm],Motor Torque RR after FW [Nm]
  Constant : Constant  Value=TV_ON
  Constant1 : Constant  Value=0
  Gain : Gain
  Gain1 : Gain
  Switch{,1..3} (4 alike) : Switch  Criteria=u2 > Threshold  SaturateOnIntegerOverflow=off  InputSameDT=off
  TV Algorithm : Subsystem  Commented=on
      settings: PortSchema="{\"entries\":[{\"content\":{\"sides\":[{\"content\":{\"connectorIds\":[\"In1\",\"In2\"]},\"type\":\"ConnectorPlacement.EquallySpacedRectSide\",\"uuid\":\"7b07616b-0ebd-48b3-9298-597f7dd07d66\"},{\"content\":{\"connectorIds\":[\"Out1\",\"Out2\"],\"side\":\"RIGHT\"},\"type\":\"ConnectorPlacement.EquallySpacedRectSide\",\"uuid\":\"1ca9a803-29a7-4f66-83a1-4b3325ff94c2\"},{\"content\":{\"connectorIds\":[\"In3\",\"In4\"],\"side\":\"TOP\"},\"type\":\"ConnectorPlacement.EquallySpacedRectSide\",\"uuid\":\"ce1bec80-9762-4372-b362-27bcbf1a4c54\"}]},\"type\":\"ConnectorPlacement.EquallySpacedConnector\",\"uuid\":\"fe6232db-ec4c-42e2-b838-1cb40525fabf\"}],\"packageUris\":[\"http://schema.mathworks.com/mf0/Connector/R2020b\"],\"version\":\"1.0\"}"
  Motor Torque after TV [Nm] : Outport
  wires:
  ? -> ABS/2(Slip_Ratio), ABS1/2(Slip_Ratio)
  Constant/1 -> Switch/2, Switch2/2, Switch3/2, Switch1/2
  Motor Torque after FW [Nm]/1 -> Bus Selector/1
  Constant1/1 -> Switch3/1, Switch2/1, Switch1/1, Switch/1
  Bus Selector/1 -> Switch/3  "<Motor Torque FL after FW [Nm]>"
  Bus Selector/2 -> Switch1/3  "<Motor Torque FR after FW [Nm]>"
  Bus Selector/3 -> Gain/1  "<Motor Torque RL after FW [Nm]>"
  Bus Selector/4 -> Gain1/1  "<Motor Torque RR after FW [Nm]>"
  Switch3/1 -> Bus Creator/4  "Motor Torque RR after TV [Nm]"
  Switch2/1 -> Bus Creator/3  "Motor Torque RL after TV [Nm]"
  Bus Creator/1 -> Motor Torque after TV [Nm]/1
  Switch/1 -> Bus Creator/1  "Motor Torque FL after TV [Nm]"
  Switch1/1 -> Bus Creator/2  "Motor Torque FR after TV [Nm]"
  Gain/1 -> Switch2/3
  Gain1/1 -> Switch3/3

== system Rebuild/Main/Powertrain/Motors/Field Weakening ==
  Requested_Motor_Torque : Inport
  Bus Creator : BusCreator  Inputs=4
  Bus Selector : BusSelector  OutputSignals=Wheel Speeds.Wheel Speeds [rad/s].Wheel Speed FL [rad/s],Wheel Speeds.Wheel Speeds [rad/s].Wheel Speed RL [rad/s],Wheel Speeds.Wheel Speeds [rad/s].Wheel Speed RR [rad/s],Wheel Speeds.Wheel Speeds [rad/s].Wheel Speed FR [rad/s]
  Constant : Constant  Value=Motor_maximum_power
  Gain : Gain  Gain=0
  Gain{1..2,5,7} (4 alike) : Gain  Gain=-1
  Gain10 : Gain
  Gain11 : Gain
  Gain{3..4,6,8} (4 alike) : Gain  Gain=Gear_ratio
  Gain9 : Gain  Gain=0
  Product : Product  Inputs=*/
  Product1 : Product  Inputs=/*
  Product2 : Product  Inputs=/*
  Product3 : Product  Inputs=*/
  Saturation Dynamic{,1..3} (4 alike) : simulink/Discontinuities/Saturation Dynamic  OutMin=[]  OutMax=[]  OutDataTypeStr=Inherit: Same as second input  OutDataType=fixdt(1, 16)  OutScaling=2^-10  DoSatur=off
  Motor Torque after FW [Nm] : Outport
  wires:
  Saturation Dynamic1/1 -> Gain10/1
  Gain2/1 -> Saturation Dynamic1/3
  Product/1 -> Gain2/1, Saturation Dynamic1/1  "Maximum Torque RR after FW [Nm]"
  Bus Selector/2 -> Gain3/1  "<Wheel Speed RL [rad/s]>"
  Gain1/1 -> Saturation Dynamic/3
  Product1/1 -> Gain1/1, Saturation Dynamic/1  "Maximum Torque RL after FW [Nm]"
  Bus Selector/3 -> Gain4/1  "<Wheel Speed RR [rad/s]>"
  Gain3/1 -> Product1/1  "Motor Speed RL [rad/s]"
  Gain4/1 -> Product/2  "Motor Speed RR [rad/s]"
  Saturation Dynamic/1 -> Gain11/1
  Saturation Dynamic2/1 -> Gain/1
  Gain6/1 -> Product2/1  "Motor Speed FL [rad/s]"
  Product2/1 -> Gain5/1, Saturation Dynamic2/1  "Maximum Torque FL after FW [Nm]"
  Bus Selector/1 -> Gain6/1  "<Wheel Speed FL [rad/s]>"
  Gain5/1 -> Saturation Dynamic2/3
  Requested_Motor_Torque/1 -> Saturation Dynamic2/2, Saturation Dynamic/2, Saturation Dynamic3/2, Saturation Dynamic1/2
  Constant/1 -> Product1/2, Product2/2, Product/1, Product3/1
  Gain8/1 -> Product3/2  "Motor Speed FR [rad/s]"
  Bus Selector/4 -> Gain8/1  "<Wheel Speed FR [rad/s]>"
  Product3/1 -> Gain7/1, Saturation Dynamic3/1  "Maximum Torque FR after FW [Nm]"
  Gain7/1 -> Saturation Dynamic3/3
  Saturation Dynamic3/1 -> Gain9/1
  [Tires] -> Bus Selector/1
  Bus Creator/1 -> Motor Torque after FW [Nm]/1
  Gain/1 -> Bus Creator/1  "Motor Torque FL after FW [Nm]"
  Gain9/1 -> Bus Creator/4  "Motor Torque FR after FW [Nm]"
  Gain10/1 -> Bus Creator/3  "Motor Torque RR after FW [Nm]"
  Gain11/1 -> Bus Creator/2  "Motor Torque RL after FW [Nm]"

== system Rebuild/Main/Powertrain/Motors/Power Limit ==
  Motor Torque after TV [Nm] : Inport
  Bus Creator : BusCreator  Inputs=4
  Bus Selector : BusSelector  OutputSignals=Motor Torque FL after TV [Nm],Motor Torque FR after TV [Nm],Motor Torque RL after TV [Nm],Motor Torque RR after TV [Nm]
  Constant : Constant  Value=TV_ON
  Constant1 : Constant  Value=0
  Power Calculation : Subsystem
  Switch{,1..3} (4 alike) : Switch  Criteria=u2 > Threshold  SaturateOnIntegerOverflow=off  InputSameDT=off
  Motor Power [W] : Outport
  Motor Torque [Nm] : Outport  Port=2
  wires:
  Motor Torque after TV [Nm]/1 -> Bus Selector/1, Power Calculation/1(In1)
  Power Calculation/1(Motor Power [W]) -> Motor Power [W]/1
  Bus Selector/2 -> Switch1/3  "<Motor Torque FR after TV [Nm]>"
  Switch3/1 -> Bus Creator/4  "Motor Torque RR [Nm]"
  Switch2/1 -> Bus Creator/3  "Motor Torque RL [Nm]"
  Switch/1 -> Bus Creator/1  "Motor Torque FL [Nm]"
  Switch1/1 -> Bus Creator/2  "Motor Torque FR [Nm]"
  Bus Selector/3 -> Switch2/3  "<Motor Torque RL after TV [Nm]>"
  Constant1/1 -> Switch3/1, Switch2/1, Switch1/1, Switch/1
  Bus Selector/4 -> Switch3/3  "<Motor Torque RR after TV [Nm]>"
  Bus Selector/1 -> Switch/3  "<Motor Torque FL after TV [Nm]>"
  Constant/1 -> Switch/2, Switch2/2, Switch3/2, Switch1/2
  Bus Creator/1 -> Motor Torque [Nm]/1

== system Rebuild/Main/Powertrain/Motors/Regen Braking ==
  Brake Pressure [bar] : Inport
  " " : Constant  Value=Front_desired_brake_p_balance
  AND : Logic  IconShape=distinctive  AllPortsSameDT=off  OutDataTypeStr=boolean
  Bus Selector : BusSelector  OutputSignals=Brake Pressure Front [bar],Brake Pressure Rear [bar]
  Cast To Boolean : DataTypeConversion  OutDataTypeStr=double  SaturateOnIntegerOverflow=off  RndMeth=Floor
  Compare To Constant : simulink/Logic and Bit Operations/Compare To Constant  relop=>=  const=5  OutDataTypeStr=boolean
  Compare To Constant1 : simulink/Logic and Bit Operations/Compare To Constant  relop=>=  const=5  OutDataTypeStr=boolean
  Gain : Gain  Gain=-1
  Product1 : Product
  Saturation2 : Saturate  UpperLimit=29  LowerLimit=0
  Subsystem : Subsystem
  Torque_to_Current_Conversion : Lookup_n-D  NumberOfTableDimensions=1  BreakpointsForDimension1=[0 29]  Table=[0 44]  InternalRulePriority=Speed  RndMeth=Simplest
  Negative Torque Command [Nm] : Outport
  wires:
  " "/1 -> Subsystem/3(Desired_Brake_Balance)  "Desired_Brake_Balance"
  Compare To Constant/1 -> AND/2
  Cast To Boolean/1 -> Product1/1
  Torque_to_Current_Conversion/1 -> Saturation2/1
  Product1/1 -> Gain/1
  Saturation2/1 -> Product1/2
  Subsystem/1("Motor_Rear_\"Preasure\"") -> Torque_to_Current_Conversion/1
  AND/1 -> Cast To Boolean/1
  Compare To Constant1/1 -> AND/1
  Brake Pressure [bar]/1 -> Bus Selector/1
  Gain/1 -> Negative Torque Command [Nm]/1  "Negative Torque Command [Nm]"
  Bus Selector/2 -> Compare To Constant/1, Subsystem/2(Brake_Preasure_Rear)  "<Brake Pressure Rear [bar]>"
  Bus Selector/1 -> Compare To Constant1/1, Subsystem/1(Brake_Preasure_Front)  "<Brake Pressure Front [bar]>"

== system Rebuild/Main/Powertrain/Motors/Torque Command [Nm] ==
  APPS : Inport
  Constant : Constant  Value=Torque_limit_set
  Merge : Merge  Inputs=11
  Switch Case : SwitchCase  CaseConditions={1,2,3,4,5,6,7,8,9,10}
  Switch Case Action Subsystem : Subsystem  TreatAsAtomicUnit=on
  Switch Case Action Subsystem1 : Subsystem  TreatAsAtomicUnit=on
  Switch Case Action Subsystem10 : Subsystem  TreatAsAtomicUnit=on
  Switch Case Action Subsystem2 : Subsystem  TreatAsAtomicUnit=on
  Switch Case Action Subsystem3 : Subsystem  TreatAsAtomicUnit=on
  Switch Case Action Subsystem4 : Subsystem  TreatAsAtomicUnit=on
  Switch Case Action Subsystem5 : Subsystem  TreatAsAtomicUnit=on
  Switch Case Action Subsystem6 : Subsystem  TreatAsAtomicUnit=on
  Switch Case Action Subsystem7 : Subsystem  TreatAsAtomicUnit=on
  Switch Case Action Subsystem8 : Subsystem  TreatAsAtomicUnit=on
  Switch Case Action Subsystem9 : Subsystem  TreatAsAtomicUnit=on
  Positive Torque Command [Nm] : Outport
  wires:
  APPS/1 -> Switch Case Action Subsystem2/1(APPS), Switch Case Action Subsystem4/1(APPS), Switch Case Action Subsystem7/1(APPS), Switch Case Action Subsystem9/1(APPS), Switch Case Action Subsystem10/1(APPS), Switch Case Action Subsystem8/1(APPS), Switch Case Action Subsystem6/1(APPS), Switch Case Action Subsystem5/1(APPS), Switch Case Action Subsystem3/1(APPS), Switch Case Action Subsystem1/1(APPS), Switch Case Action Subsystem/1(APPS)
  Switch Case/2 -> Switch Case Action Subsystem9/Action
  Switch Case Action Subsystem8/1(Out1) -> Merge/3
  Switch Case/1 -> Switch Case Action Subsystem10/Action
  Merge/1 -> Positive Torque Command [Nm]/1
  Switch Case Action Subsystem1/1(Out1) -> Merge/10
  Switch Case/9 -> Switch Case Action Subsystem2/Action
  Switch Case Action Subsystem7/1(Out1) -> Merge/4
  Switch Case/7 -> Switch Case Action Subsystem4/Action
  Constant/1 -> Switch Case/1
  Switch Case/11 -> Switch Case Action Subsystem/Action
  Switch Case Action Subsystem9/1(Out1) -> Merge/2
  Switch Case Action Subsystem10/1(Out1) -> Merge/1
  Switch Case Action Subsystem6/1(Out1) -> Merge/5
  Switch Case Action Subsystem4/1(Out1) -> Merge/7
  Switch Case Action Subsystem3/1(Out1) -> Merge/8
  Switch Case/6 -> Switch Case Action Subsystem5/Action
  Switch Case Action Subsystem5/1(Out1) -> Merge/6
  Switch Case Action Subsystem2/1(Out1) -> Merge/9
  Switch Case Action Subsystem/1(Out1) -> Merge/11
  Switch Case/10 -> Switch Case Action Subsystem1/Action
  Switch Case/5 -> Switch Case Action Subsystem6/Action
  Switch Case/4 -> Switch Case Action Subsystem7/Action
  Switch Case/3 -> Switch Case Action Subsystem8/Action
  Switch Case/8 -> Switch Case Action Subsystem3/Action

== system Rebuild/Main/Wheels & Tires/Brakes/Brake_Balance_Adjustment ==
  Braking_Torque_F [Nm] : Inport
  Braking_Torque_R [Nm] : Inport  Port=2
  Add : Sum
  Add1 : Sum
  Add2 : Sum
  Compare To Constant1 : simulink/Logic and Bit Operations/Compare To Constant  relop=>  const=1  OutDataTypeStr=boolean
  Constant : Constant  Value=Lock_brake_balance
  Constant1 : Constant  Value=Lock_brake_balance
  Constant2 : Constant  Value=Front_brake_balance
  Enabled Subsystem : Subsystem  TreatAsAtomicUnit=on
  Product : Product  Inputs=*/
  Product1 : Product
  Subtract : Sum  Inputs=-+
  Subtract1 : Sum  Inputs=-+
  Switch : Switch  Threshold=1  SaturateOnIntegerOverflow=off  InputSameDT=off
  Switch1 : Switch  Threshold=1  SaturateOnIntegerOverflow=off  InputSameDT=off
  Terminator : Terminator
  Adj_Braking_Torque_F [Nm] : Outport
  Adj_Braking_Torque_R [Nm] : Outport  Port=2
  wires:
  Constant/1 -> Switch/2
  Switch/1 -> Adj_Braking_Torque_F [Nm]/1, Product/1, Add/1  "Adj_Front"
  Switch1/1 -> Add/2, Compare To Constant1/1, Adj_Braking_Torque_R [Nm]/1  "Adj_Rear"
  Constant1/1 -> Switch1/2
  Add/1 -> Product/2
  Product/1 -> Enabled Subsystem/1(In1)  "Brake_balance"
  Enabled Subsystem/1(Out1) -> Terminator/1  "Brake_balance"
  Compare To Constant1/1 -> Enabled Subsystem/Enable
  Constant2/1 -> Product1/1
  Braking_Torque_F [Nm]/1 -> Add1/1, Add2/1
  Product1/1 -> Subtract1/1, Subtract/1, Add1/2, Switch/1  "Adjusted_Torque_F"
  Braking_Torque_R [Nm]/1 -> Add2/2, Subtract/2
  Add2/1 -> Product1/2, Subtract1/2
  Subtract1/1 -> Switch1/1  "Adjusted_Torque_R"
  Add1/1 -> Switch/3  "Locked_Torque_F"
  Subtract/1 -> Switch1/3  "Locked_Torque_R"

== system Rebuild/Main/Wheels & Tires/Brakes/Braking_Torque_Front ==
  Brake_Pressure [bar] : Inport
  Gain : Gain  Gain=1e5
  Gain1 : Gain  Gain=Effective_br_disk_r_F
  Product : Product  Inputs=3
  coefficient of friction : Constant  Value=Br_coef_of_friction_F
  piston area : Constant  Value=Br_pistons_area_F
  Braking_torque [Nm] : Outport
  wires:
  Brake_Pressure [bar]/1 -> Gain/1  "[bar]"
  Gain/1 -> Product/1  "[Pa]"
  coefficient of friction/1 -> Product/2
  piston area/1 -> Product/3
  Product/1 -> Gain1/1  "Braking force [N]"
  Gain1/1 -> Braking_torque [Nm]/1  "Braking torque [Nm]"

== system Rebuild/Main/Wheels & Tires/Brakes/Braking_Torque_Rear ==
  Brake_Pressure [bar] : Inport
  Gain1 : Gain  Gain=1e5
  Gain2 : Gain  Gain=Effective_br_disk_r_R
  Product2 : Product  Inputs=3
  coefficient of friction : Constant  Value=Br_coef_of_friction_R
  piston area : Constant  Value=Br_pistons_area_R
  Braking_Torque [Nm] : Outport
  wires:
  Product2/1 -> Gain2/1  "Braking_Force [N]"
  piston area/1 -> Product2/3
  Gain2/1 -> Braking_Torque [Nm]/1  "Braking_Torque [Nm]"
  Gain1/1 -> Product2/1  "[Pa]"
  coefficient of friction/1 -> Product2/2
  Brake_Pressure [bar]/1 -> Gain1/1

== system Rebuild/Main/Wheels & Tires/Slip Ratio & Slip Angle Calculation/Slip Angle ==
  Bus Creator : BusCreator  Inputs=4
  Bus Selector : BusSelector  OutputSignals=Steering Angle [rad].Steering Angle FL [rad]
  Bus Selector1 : BusSelector  OutputSignals=Velocitiy [m/s].X Velocity [m/s],Velocitiy [m/s].Y Velocity [m/s],Velocitiy [m/s].Yaw_Rate [rad/s]
  Bus Selector3 : BusSelector  OutputSignals=Steering Angle [rad].Steering Angle FR [rad]
  Bus Selector4 : BusSelector  OutputSignals=Steering Angle [rad].Steering Angle RL [rad]
  Bus Selector5 : BusSelector  OutputSignals=Steering Angle [rad].Steering Angle RR [rad]
  Slip Angle FL : Subsystem
  Slip Angle FR : Subsystem
  Slip Angle RL : Subsystem
  Slip Angle RR : Subsystem
  Slip Angle [rad] : Outport
  wires:
  [Sus] -> Bus Selector5/1, Bus Selector4/1, Bus Selector3/1, Bus Selector/1
  Bus Selector/1 -> Slip Angle FL/4(Steering Angle FL [rad])  "<Steering Angle FL [rad]>"
  Bus Creator/1 -> Slip Angle [rad]/1
  Slip Angle FL/1(Slip Angle FL [rad]) -> Bus Creator/1  "Slip Angle FL [rad]"
  Slip Angle FR/1(Slip Angle FR [rad]) -> Bus Creator/2  "Slip Angle FR [rad]"
  Slip Angle RL/1(Slip Angle RL [rad]) -> Bus Creator/3  "Slip Angle RL [rad]"
  Slip Angle RR/1(Slip Angle RR [rad]) -> Bus Creator/4  "Slip Angle RR [rad]"
  [States] -> Bus Selector1/1
  Bus Selector1/1 -> Slip Angle FL/1(X Velocity [m/s]), Slip Angle RR/1(X Velocity [m/s]), Slip Angle RL/1(X Velocity [m/s]), Slip Angle FR/1(X Velocity [m/s])  "<X Velocity [m/s]>"
  Bus Selector1/2 -> Slip Angle FL/2(Y Velocity [m/s]), Slip Angle FR/2(Y Velocity [m/s]), Slip Angle RR/2(Y Velocity [m/s]), Slip Angle RL/2(Y Velocity [m/s])  "<Y Velocity [m/s]>"
  Bus Selector1/3 -> Slip Angle FL/3(Yaw Rate [rad/s]), Slip Angle RR/3(Yaw Rate [rad/s]), Slip Angle RL/3(Yaw Rate [rad/s]), Slip Angle FR/3(Yaw Rate [rad/s])  "<Yaw_Rate [rad/s]>"
  Bus Selector3/1 -> Slip Angle FR/4(Steering Angle FR [rad])  "<Steering Angle FR [rad]>"
  Bus Selector4/1 -> Slip Angle RL/4(Steering Angle RL [rad])  "<Steering Angle RL [rad]>"
  Bus Selector5/1 -> Slip Angle RR/4(Steering Angle RR [rad])  "<Steering Angle RR [rad]>"

== system Rebuild/Main/Wheels & Tires/Slip Ratio & Slip Angle Calculation/Slip Ratio  ==
  Wheel Speeds [rad/s] : Inport
  Bus Creator : BusCreator  Inputs=4
  Bus Selector : BusSelector  OutputSignals=Wheel Speeds [rad/s].Wheel Speed FL [rad/s],Wheel Speeds [rad/s].Wheel Speed FR [rad/s],Wheel Speeds [rad/s].Wheel Speed RL [rad/s],Wheel Speeds [rad/s].Wheel Speed RR [rad/s]
  Bus Selector1 : BusSelector  OutputSignals=Velocitiy [m/s].X Velocity [m/s]
  Slip ratio FL : Subsystem
  Slip ratio FR : Subsystem
  Slip ratio RL : Subsystem
  Slip ratio RR : Subsystem
  Slip Ratio : Outport
  wires:
  Wheel Speeds [rad/s]/1 -> Bus Selector/1
  Bus Creator/1 -> Slip Ratio/1
  Bus Selector/1 -> Slip ratio FL/1(Wheel Speed FL [rad/s])  "<Wheel Speed FL [rad/s]>"
  Bus Selector/2 -> Slip ratio FR/1(Wheel Speed FR [rad/s])  "<Wheel Speed FR [rad/s]>"
  Bus Selector/3 -> Slip ratio RL/1(Wheel Speed RL [rad/s])  "<Wheel Speed RL [rad/s]>"
  Bus Selector/4 -> Slip ratio RR/1(Wheel Speed RR [rad/s])  "<Wheel Speed RR [rad/s]>"
  Slip ratio FL/1(Slip Ratio FL) -> Bus Creator/1  "Slip Ratio FL"
  Slip ratio FR/1(Slip Ratio FR) -> Bus Creator/2  "Slip Ratio FR"
  Slip ratio RL/1(Slip Ratio RL) -> Bus Creator/3  "Slip Ratio RL"
  Slip ratio RR/1(Slip Ratio RR) -> Bus Creator/4  "Slip Ratio RR"
  Bus Selector1/1 -> Slip ratio FR/2(X Velocity [m/s]), Slip ratio RL/2(X Velocity [m/s]), Slip ratio RR/2(X Velocity [m/s]), Slip ratio FL/2(X Velocity [m/s])  "<X Velocity [m/s]>"
  [States] -> Bus Selector1/1

== system Rebuild/Main/Wheels & Tires/Wheel Speeds/Rolling Resistance Calculation ==
  Fz [N] : Inport
  Bus Selector : BusSelector  OutputSignals=Fz FL [N],Fz FR [N],Fz RL [N],Fz RR [N]
  Bus Creator : BusCreator  Inputs=4
  Gain{,1,4,6} (4 alike) : Gain  Gain=Tire_radius
  Gain{2..3,5,7} (4 alike) : Gain  Gain=Wheel_rolling_resistance
  Rolling Resistance : Outport
  wires:
  Gain/1 -> Gain2/1
  Gain2/1 -> Bus Creator/1  "Rolling Resistance FL"
  Gain3/1 -> Bus Creator/2  "Rolling Resistance FR"
  Gain5/1 -> Bus Creator/3  "Rolling Resistance RL"
  Gain7/1 -> Bus Creator/4  "Rolling Resistance RR"
  Bus Creator/1 -> Rolling Resistance/1  "Rolling Resistance"
  Fz [N]/1 -> Bus Selector/1
  Bus Selector/1 -> Gain/1  "<Fz FL [N]>"
  Gain1/1 -> Gain3/1
  Gain4/1 -> Gain5/1
  Gain6/1 -> Gain7/1
  Bus Selector/2 -> Gain1/1  "<Fz FR [N]>"
  Bus Selector/3 -> Gain4/1  "<Fz RL [N]>"
  Bus Selector/4 -> Gain6/1  "<Fz RR [N]>"

== system Rebuild/Main/Wheels & Tires/Wheel Speeds/Wheel Speed FL ==
  Rolling Resistance : Inport
  Fx [N] : Inport  Port=2
  Torque [Nm] : Inport  Port=3
  Add1 : Sum  Inputs=--+-
  Bus Selector : BusSelector  OutputSignals=Brake Torque [Nm].Brake Torque FL [Nm],Motor Torque [Nm].Motor Torque FL [Nm]
  Bus Selector1 : BusSelector  OutputSignals=Rolling Resistance FL
  Bus Selector2 : BusSelector  OutputSignals=Fx FL [N]
  Constant4 : Constant  Value=Tire_radius
  Gain : Gain  Gain=Gear_ratio
  Gain1 : Gain  Gain=1/Iz_wheel
  Integrator2 : Integrator  InitialCondition=start_velocity_x / Tire_radius
  Product : Product
  Saturation : Saturate  UpperLimit=200  LowerLimit=-20
  Wheel Speed FL [rad/s] : Outport
  wires:
  Bus Selector/2 -> Gain/1  "<Motor Torque FL [Nm]>"
  Add1/1 -> Gain1/1
  Integrator2/1 -> Saturation/1
  Gain1/1 -> Integrator2/1
  Bus Selector2/1 -> Product/2  "<Fx FL [N]>"
  Fx [N]/1 -> Bus Selector2/1
  Bus Selector/1 -> Add1/2  "<Brake Torque FL [Nm]>"
  Bus Selector1/1 -> Add1/4  "<Rolling Resistance FL>"
  Constant4/1 -> Product/1
  Product/1 -> Add1/1
  Torque [Nm]/1 -> Bus Selector/1
  Rolling Resistance/1 -> Bus Selector1/1
  Saturation/1 -> Wheel Speed FL [rad/s]/1
  Gain/1 -> Add1/3

== system Rebuild/Main/Wheels & Tires/Wheel Speeds/Wheel Speed FR ==
  Rolling Resistance : Inport
  Fx [N] : Inport  Port=2
  Torque [Nm] : Inport  Port=3
  Add1 : Sum  Inputs=--+-
  Bus Selector : BusSelector  OutputSignals=Brake Torque [Nm].Brake Torque FR [Nm],Motor Torque [Nm].Motor Torque FR [Nm]
  Bus Selector1 : BusSelector  OutputSignals=Rolling Resistance RL
  Bus Selector2 : BusSelector  OutputSignals=Fx FR [N]
  Constant4 : Constant  Value=Tire_radius
  Gain : Gain  Gain=Gear_ratio
  Gain1 : Gain  Gain=1/Iz_wheel
  Integrator2 : Integrator  InitialCondition=start_velocity_x / Tire_radius
  Product : Product
  Saturation : Saturate  UpperLimit=200  LowerLimit=-20
  Wheel Speed FR [rad/s] : Outport
  wires:
  Bus Selector/2 -> Gain/1  "<Motor Torque FR [Nm]>"
  Add1/1 -> Gain1/1
  Integrator2/1 -> Saturation/1
  Gain1/1 -> Integrator2/1
  Bus Selector2/1 -> Product/2  "<Fx FR [N]>"
  Fx [N]/1 -> Bus Selector2/1
  Bus Selector/1 -> Add1/2  "<Brake Torque FR [Nm]>"
  Bus Selector1/1 -> Add1/4  "<Rolling Resistance RL>"
  Constant4/1 -> Product/1
  Product/1 -> Add1/1
  Torque [Nm]/1 -> Bus Selector/1
  Rolling Resistance/1 -> Bus Selector1/1
  Saturation/1 -> Wheel Speed FR [rad/s]/1
  Gain/1 -> Add1/3
